simulink model "lqr_identification"  (R2017a)
settings: Solver=ode5  StartTime=0.0  StopTime=50  FixedStep=Ts  RelTol=1e-3  EnableMultiTasking=on
values from neighbouring files (symbols this model uses):
  B_ENU_inv = pinv(B_ENU)    [firefly_param_test.m]
  gra = 9.80665    [firefly_param_test.m]
  Ki_lqr = [0 0 0.1 0 0 -0.1 0 0 8.66025403784 0 0 0 ... (16 elements, 4x4)]    [K_lqr_tracking_ENU.mat]
  KT = 0.00000854858    (= 8.54858e-06)    [firefly_param_test.m]
  Kx_lqr = [0 0 0.263619393691 0 0 -0.257300038922 0 0 13.6588017709 0 0 0 ... (48 elements, 4x12)]    [K_lqr_tracking_ENU.mat]
  mass = 1.49    [firefly_param_test.m]
settings Model: Creator=dtnguyen  LastModifiedBy=ducnguyen
settings DataIOCC: LimitDataPoints=on  SaveFormat=Array
settings OptimizationCC: DefaultParameterBehavior=Inlined  UseFloatMulNetSlope=on  InlineInvariantSignals=on  PassReuseOutputArgsThreshold=0  EfficientFloat2IntCast=on
settings DebuggingCC: ParameterTunabilityLossMsg=error  SFUnexpectedBacktrackingDiag=warning  SFNoUnconditionalDefaultTransitionDiag=warning  SFExecutionAtInitializationDiag=none
settings HardwareCC: ProdBitPerPointer=32  ProdBitPerSizeT=32  ProdBitPerPtrDiffT=32  ProdLargestAtomicFloat=None  ProdIntDivRoundTo=Undefined  ProdEndianess=Unspecified  ProdWordSize=32  ProdHWDeviceType=32-bit Generic
settings ModelReferenceCC: PropagateSignalLabelsOutOfModel=off
settings RTWCC: PackageName=myCodeExport  GenerateReport=on  Toolchain=Catkin  BuildConfiguration=Faster Runs  LaunchReport=on  TargetLang=C++  CheckMdlBeforeBuild=Warning
settings CodeAppCC: ForceParamTrailComments=on  OperatorAnnotations=on  MATLABSourceComments=on
settings GRTTargetCC: TargetLangStandard=C++03 (ISO)  MatFileLogging=off  MultiInstanceERTCode=on  CodeInterfacePackaging=C++ class
settings ConfigComp: CovMetricSettings=dw  CovHtmlReporting=on  CovSaveCumulativeToWorkspaceVar=on  CovSaveSingleToWorkspaceVar=on  CovExternalEMLEnable=off

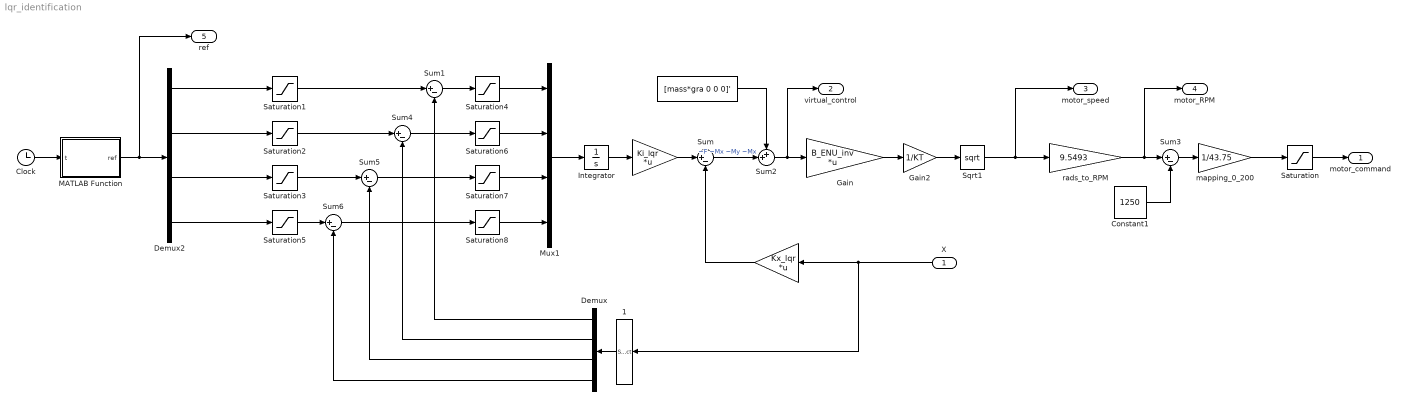
== system lqr_identification ==
  X : Inport  PortDimensions=12
  " " : Gain  Gain=Ki_lqr  Multiplication=Matrix(K*u)
  "              " : Constant  Value=[mass*gra 0 0 0]'
  "                   " : Gain  Gain=Kx_lqr  Multiplication=Matrix(K*u)
  "                    1" : Selector  InputPortWidth=12  IndexOptions=Index vector (dialog)  Indices=[1 2 3 9]  OutputSizes=1
  Clock : Clock
  Constant1 : Constant  Value=1250  VectorParams1D=off  SampleTime=-1
  Demux : Demux
  Demux2 : Demux
  Gain : Gain  Gain=B_ENU_inv  Multiplication=Matrix(K*u)
  Gain2 : Gain  Gain=1/KT
  Integrator : Integrator  InitialCondition=[0 0 0 0]'
  MATLAB Function : MATLAB Function  TreatAsAtomicUnit=on
  Mux1 : Mux
  Saturation : Saturate  UpperLimit=200  LowerLimit=0
  Saturation{1..2,4,6} (4 alike) : Saturate  UpperLimit=1  LowerLimit=-1
  Saturation3 : Saturate  UpperLimit=1  LowerLimit=0
  Saturation5 : Saturate  UpperLimit=2*pi  LowerLimit=-2*pi
  Saturation7 : Saturate
  Saturation8 : Saturate  UpperLimit=pi/4  LowerLimit=-pi/4
  Sqrt1 : Sqrt  SaturateOnIntegerOverflow=on
  Sum{,1,3..6} (6 alike) : Sum  Inputs=|+-
  Sum2 : Sum  Inputs=++|
  mapping_0_200 : Gain  Gain=1/43.75
  rads_to_RPM : Gain  Gain=9.5493
  motor_command : Outport  PortDimensions=6
  virtual_control : Outport  Port=2  PortDimensions=4
  motor_speed : Outport  Port=3  PortDimensions=6
  motor_RPM : Outport  Port=4  PortDimensions=6
  ref : Outport  Port=5  PortDimensions=4
  wires:
  Gain2/1 -> Sqrt1/1
  X/1 -> "                   "/1, "                    1"/1
  Mux1/1 -> Integrator/1
  " "/1 -> Sum/1
  Integrator/1 -> " "/1
  "                   "/1 -> Sum/2
  Gain/1 -> Gain2/1
  Sum2/1 -> Gain/1, virtual_control/1
  Constant1/1 -> Sum3/2
  rads_to_RPM/1 -> Sum3/1, motor_RPM/1
  Sum3/1 -> mapping_0_200/1
  mapping_0_200/1 -> Saturation/1
  Saturation/1 -> motor_command/1
  Saturation1/1 -> Sum1/1
  Sum1/1 -> Saturation4/1
  Sum4/1 -> Saturation6/1
  Sum5/1 -> Saturation7/1
  Sum6/1 -> Saturation8/1
  "                    1"/1 -> Demux/1
  Demux/1 -> Sum1/2
  Demux/2 -> Sum4/2
  Demux/3 -> Sum5/2
  Demux/4 -> Sum6/2
  Saturation2/1 -> Sum4/1
  Saturation3/1 -> Sum5/1
  Saturation4/1 -> Mux1/1
  Saturation5/1 -> Sum6/1
  Saturation6/1 -> Mux1/2
  Saturation7/1 -> Mux1/3
  Saturation8/1 -> Mux1/4
  Sqrt1/1 -> rads_to_RPM/1, motor_speed/1
  Demux2/3 -> Saturation3/1
  Demux2/2 -> Saturation2/1
  Clock/1 -> MATLAB Function/1(t)
  MATLAB Function/1(ref) -> Demux2/1, ref/1
  Demux2/1 -> Saturation1/1
  Sum/1 -> Sum2/2  "~F ~Mx ~My ~Mx"
  "              "/1 -> Sum2/1
  Demux2/4 -> Saturation5/1

== matlab function lqr_identification/MATLAB Function ==
  data: t input; ref output
function ref = fcn(t)
x = 0; y = 0; z = 0;psi = 0;
if t <= 20
    x = 0;
    y = 0; 
    z = 0.5;
    psi = 0;
elseif t <= 40
    x = -1;
    y = 0;
    z = 0.5;
    psi = 0;
elseif t <= 60
    x = -1;
    y = 1;
    z = 0.5;
    psi = 0;
elseif t <= 90
    x = -1;
    y = 1;
    z = 0.5;
    psi = pi/6;
else
    x = -1;
    y = 1;
    z = 0;
    psi = 0;
end
ref = [x;y;z;psi];
